simulink model "xieboduoji_13fangzhennow"  (R2023a)
settings: Solver=ode4  StartTime=0.0  StopTime=2.2  FixedStep=5e-7  RelTol=1e-3
undefined symbols (not defined in the file or in its folder): magnitude
libraries: simulink x417, spsRMSLib x70, spsCurrentMeasurementLib x32, spsVoltageMeasurementLib x31, powerlib_meascontrol x24, spsFourierLib x21, spsGroundLib x19, spsThreePhasePISectionLineLib x17, spsThreePhaseSeriesRLCBranchLib x14, spsdq0toAlphaBetaZeroLib x13, spsSeriesRLCBranchLib x11, spsUniversalBridgeLib x11
(part 2 of 12)

== system xieboduoji_13fangzhennow/node10/Subsystem2 ==
  u1 : Inport
  u3 : Inport  Port=2
  u4 : Inport  Port=3
  u5 : Inport  Port=4
  u6 : Inport  Port=5
  u2 : Inport  Port=6
  Pul : DiscretePulseGenerator  PulseType=Time based  Period=5e-5  PulseWidth=40
  RMS1 : Subsystem  TreatAsAtomicUnit=on
  k1 : Outport  VectorParamsAs1DForOutWhenUnconnected=off
  k2 : Outport  Port=2  VectorParamsAs1DForOutWhenUnconnected=off
  k3 : Outport  Port=3  VectorParamsAs1DForOutWhenUnconnected=off
  k4 : Outport  Port=4  VectorParamsAs1DForOutWhenUnconnected=off
  k5 : Outport  Port=5  VectorParamsAs1DForOutWhenUnconnected=off
  k6 : Outport  Port=6  VectorParamsAs1DForOutWhenUnconnected=off
  k7 : Outport  Port=7  VectorParamsAs1DForOutWhenUnconnected=off
  k8 : Outport  Port=8  VectorParamsAs1DForOutWhenUnconnected=off
  k9 : Outport  Port=9  VectorParamsAs1DForOutWhenUnconnected=off
  k10 : Outport  Port=10  VectorParamsAs1DForOutWhenUnconnected=off
  k11 : Outport  Port=11  VectorParamsAs1DForOutWhenUnconnected=off
  k12 : Outport  Port=12  VectorParamsAs1DForOutWhenUnconnected=off
  wires:
  Pul/1 -> RMS1/Trigger
  RMS1/1(k1) -> k1/1
  RMS1/2(k2) -> k2/1
  RMS1/3(k3) -> k3/1
  RMS1/4(k4) -> k4/1
  RMS1/5(k5) -> k5/1
  RMS1/6(k6) -> k6/1
  RMS1/7(k7) -> k7/1
  RMS1/8(k8) -> k8/1
  RMS1/9(k9) -> k9/1
  RMS1/10(k10) -> k10/1
  RMS1/11(k11) -> k11/1
  RMS1/12(k12) -> k12/1
  u1/1 -> RMS1/1(u1)
  u3/1 -> RMS1/2(u3)
  u4/1 -> RMS1/3(u4)
  u5/1 -> RMS1/4(u5)
  u6/1 -> RMS1/5(u6)
  u2/1 -> RMS1/6(u2)

== system xieboduoji_13fangzhennow/node10/谐波源 ==
  Current Measurement1 : spsCurrentMeasurementLib/Current Measurement  PhasorSimulation=off  OutputType=Complex  PSBequivalent=0
  Demux1 : Demux  Commented=on  Outputs=6
  Demux2 : Demux  Commented=on  Outputs=6
  Display{,1..23} (24 alike) : Display  Commented=on
  Scope : Scope  Commented=on
  Scope1 : Scope  Commented=on
  Series RLC Branch3 : spsSeriesRLCBranchLib/Series RLC Branch  LConnTagsString=__new0  RConnTagsString=__new0  BranchType=R  Resistance=33.94  Inductance=0.5e-3  SetiL0=off  InitialCurrent=0  Capacitance=1e-6  Setx0=off  InitialVoltage=0  Measurements=None
  Subsystem1 : Subsystem  Commented=on
  Subsystem2 : Subsystem  Commented=on
  Universal Bridge : spsUniversalBridgeLib/Universal Bridge  Arms=3  SnubberResistance=1e5  SnubberCapacitance=inf  Device=Diodes  Ron=1e-3  Lon=0  ForwardVoltages="[  0  0  ]"  ForwardVoltage=0  GTOparameters=[ 10e-6 , 20e-6 ]  IGBTparameters=[ 1e-6 , 2e-6 ]  Measurements=None  Measurements_2=None  converterType=Rectifier
  傅里叶分解 : spsFourierLib/Fourier  Commented=on  Freq=50  n=[5 7 11 13 17 19]  InInit=[0, 0]  Ts=0
  A : PMIOPort  Side=Left
  B : PMIOPort  Port=2  Side=Left
  C : PMIOPort  Port=3  Side=Left
  wires:
  傅里叶分解/1 -> Demux1/1, Scope/1
  傅里叶分解/2 -> Demux2/1, Scope1/1
  Current Measurement1/1 -> 傅里叶分解/1
  Subsystem2/5(k5) -> Display4/1
  Subsystem2/2(k2) -> Display1/1
  Subsystem2/12(k12) -> Display11/1
  Subsystem2/9(k9) -> Display8/1
  Subsystem2/8(k8) -> Display7/1
  Subsystem1/1(k1) -> Display12/1
  Subsystem1/7(k7) -> Display20/1
  Subsystem1/10(k10) -> Display23/1
  Subsystem1/3(k3) -> Display16/1
  Subsystem1/5(k5) -> Display18/1
  Subsystem2/11(k11) -> Display10/1
  Subsystem1/9(k9) -> Display22/1
  Subsystem1/11(k11) -> Display14/1
  Subsystem1/6(k6) -> Display19/1
  Subsystem1/2(k2) -> Display13/1
  Subsystem1/4(k4) -> Display17/1
  Subsystem1/12(k12) -> Display15/1
  Demux2/5 -> Subsystem1/5(u6)
  Demux2/4 -> Subsystem1/4(u5)
  Demux2/2 -> Subsystem1/2(u3)
  Demux2/6 -> Subsystem1/6(u2)
  Demux2/1 -> Subsystem1/1(u1)
  Subsystem2/6(k6) -> Display5/1
  Subsystem2/4(k4) -> Display3/1
  Subsystem2/7(k7) -> Display6/1
  Demux1/6 -> Subsystem2/6(u2)
  Demux1/5 -> Subsystem2/5(u6)
  Demux1/2 -> Subsystem2/2(u3)
  Demux1/4 -> Subsystem2/4(u5)
  Subsystem1/8(k8) -> Display21/1
  Subsystem2/10(k10) -> Display9/1
  Demux1/3 -> Subsystem2/3(u4)
  Subsystem2/3(k3) -> Display2/1
  Demux1/1 -> Subsystem2/1(u1)
  Demux2/3 -> Subsystem1/3(u4)
  Subsystem2/1(k1) -> Display/1
  connections:
  Universal Bridge/LConn3 -- C/RConn1
  Universal Bridge/RConn2 -- Series RLC Branch3/RConn1
  Universal Bridge/RConn1 -- Series RLC Branch3/LConn1
  Universal Bridge/LConn2 -- B/RConn1
  Current Measurement1/LConn1 -- Universal Bridge/LConn1
  A/RConn1 -- Current Measurement1/RConn1

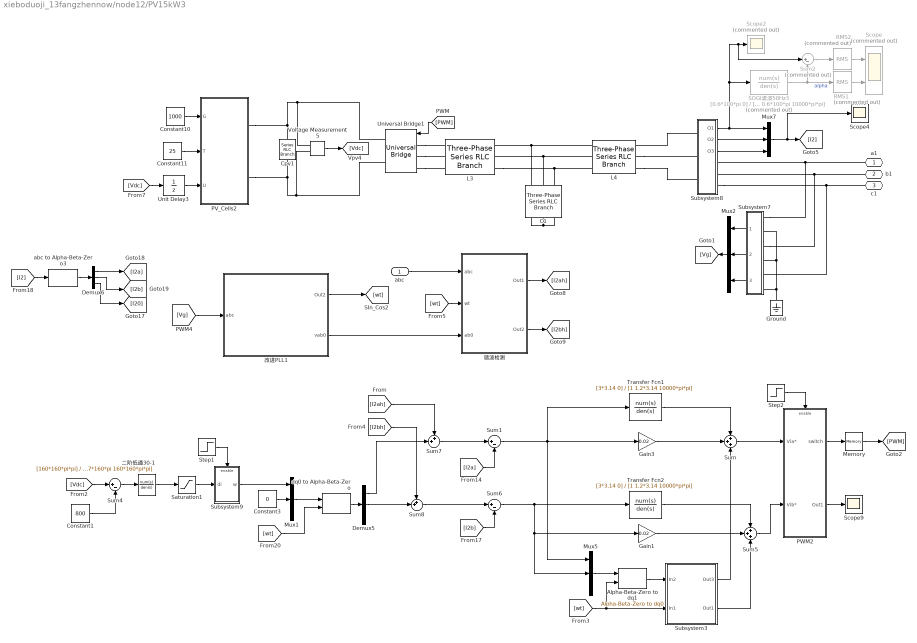
== system xieboduoji_13fangzhennow/node12/PV15kW3 ==
  abc : Inport
  " 二阶低通30-1" : TransferFcn  Numerator=[160*160*pi*pi]  Denominator=[1 2*0.707*160*pi 160*160*pi*pi]
  Alpha-Beta-Zero to dq1 : spsAlphaBetaZerotodq0Lib/Alpha-Beta-Zero to dq0  Alignment=90 degrees behind phase A axis
  C1 : spsThreePhaseSeriesRLCBranchLib/Three-Phase Series RLC Branch  LConnTagsString=A|B|C  RConnTagsString=A|B|C  BranchType=RC  Resistance=6  Inductance=1.5e-3  Capacitance=3e-6  Measurements=None
  Constant1 : Constant  Value=800
  Constant10 : Constant  Value=1000
  Constant11 : Constant  Value=25
  Constant3 : Constant  Value=0
  Cpv1 : spsSeriesRLCBranchLib/Series RLC Branch  LConnTagsString=__new0  RConnTagsString=__new0  BranchType=C  Resistance=0.2  Inductance=0.01e-3  SetiL0=off  InitialCurrent=0  Capacitance=2.5e-3  Setx0=on  InitialVoltage=800  Measurements=None
  Demux5 : Demux  Outputs=3
  Demux6 : Demux  Outputs=3
  Gain1 : Gain  Gain=0.02
  Gain3 : Gain  Gain=0.02
  Ground : spsGroundLib/Ground  LConnTagsString=a
  L3 : spsThreePhaseSeriesRLCBranchLib/Three-Phase Series RLC Branch  LConnTagsString=A|B|C  RConnTagsString=A|B|C  BranchType=L  Resistance=0.02  Inductance=2e-3  Capacitance=1e-6  Measurements=None
  L4 : spsThreePhaseSeriesRLCBranchLib/Three-Phase Series RLC Branch  LConnTagsString=A|B|C  RConnTagsString=A|B|C  BranchType=L  Resistance=0.02  Inductance=0.2e-3  Capacitance=1e-6  Measurements=None
  Memory : Memory
  Mux{1..2,5,7} (4 alike) : Mux  Inputs=3
  PV_Cells2 : Subsystem  mask{Parallel=1.6476, Series=30.3474}
  PWM2 : Subsystem
  RMS1 : spsRMSLib/RMS  Commented=on  TrueRMS=on  Freq=50  RMSInit=0  Ts=5e-5
  RMS2 : spsRMSLib/RMS  Commented=on  TrueRMS=on  Freq=50  RMSInit=0  Ts=5e-5
  SOGI滤波50Hz3 : TransferFcn  Commented=on  Numerator=[0.6*100*pi 0]  Denominator=[1 0.6*100*pi 10000*pi*pi]
  Saturation1 : Saturate  UpperLimit=15  LowerLimit=-15
  Scope : Scope  Commented=on  NumInputPorts=2
  Scope2 : Scope  Commented=on
  Scope4 : Scope
  Scope9 : Scope
  Step1 : Step  Time=0.4  SampleTime=0
  Step2 : Step  Time=0.4  SampleTime=0
  Subsystem3 : Subsystem
  Subsystem7 : Subsystem
  Subsystem8 : Subsystem
  Subsystem9 : Subsystem
  Sum : Sum  Inputs=+++
  Sum1 : Sum  Inputs=|+-
  Sum2 : Sum  Commented=on  Inputs=|+-
  Sum4 : Sum  Inputs=|+-
  Sum5 : Sum  Inputs=+++
  Sum6 : Sum  Inputs=|+-
  Sum7 : Sum  Inputs=++|
  Sum8 : Sum  Inputs=++|
  Transfer Fcn1 : TransferFcn  Numerator=[3*3.14 0]  Denominator=[1 1.2*3.14 10000*pi*pi]
  Transfer Fcn2 : TransferFcn  Numerator=[3*3.14 0]  Denominator=[1 1.2*3.14 10000*pi*pi]
  Unit Delay3 : UnitDelay  SampleTime=-1  HasFrameUpgradeWarning=on
  Universal Bridge1 : spsUniversalBridgeLib/Universal Bridge  Arms=3  SnubberResistance=1e5  SnubberCapacitance=inf  Device=IGBT / Diodes  Ron=0.002  Lon=0  ForwardVoltages="[  0  0  ]"  ForwardVoltage=0  GTOparameters=[ 10e-6 , 20e-6 ]  IGBTparameters=[ 1e-6 , 2e-6 ]  Measurements=None  Measurements_2=None  converterType=Rectifier
  Voltage Measurement5 : spsVoltageMeasurementLib/Voltage Measurement  PhasorSimulation=off  OutputType=Complex  PSBequivalent=0
  abc to Alpha-Beta-Zero3 : spsabctoAlphaBetaZeroLib/abc to Alpha-Beta-Zero
  dq0 to Alpha-Beta-Zero : spsdq0toAlphaBetaZeroLib/dq0 to Alpha-Beta-Zero  Alignment=Aligned with phase A axis
  改进PLL1 : Subsystem
  谐波检测 : Subsystem
  a1 : PMIOPort  Side=Right
  b1 : PMIOPort  Port=2  Side=Right
  c1 : PMIOPort  Port=3  Side=Right
  wires:
  Memory/1 -> [PWM]
  PWM2/2(Out1) -> Scope9/1
  Mux7/1 -> Scope4/1, [I2]
  [PWM] -> Universal Bridge1/1
  Subsystem8/3(O3) -> Mux7/3
  Subsystem8/2(O2) -> Mux7/2
  PWM2/1(switch) -> Memory/1
  Mux2/1 -> [Vg]
  Subsystem8/1(O1) -> Sum2/1, Scope2/1, SOGI滤波50Hz3/1, Mux7/1
  Subsystem7/1(O1) -> Mux2/1
  Subsystem7/2(O2) -> Mux2/2
  Subsystem7/3(O3) -> Mux2/3
  [I2b] -> Sum6/2
  Sum4/1 -> " 二阶低通30-1"/1
  Constant1/1 -> Sum4/2
  Mux1/1 -> dq0 to Alpha-Beta-Zero/1
  Sum1/1 -> Gain3/1, Transfer Fcn1/1, Mux5/1
  [wt] -> dq0 to Alpha-Beta-Zero/2
  dq0 to Alpha-Beta-Zero/1 -> Demux5/1
  Sum6/1 -> Gain1/1, Mux5/2, Transfer Fcn2/1
  [I2a] -> Sum1/2
  Sum7/1 -> Sum1/1
  Demux5/1 -> Sum7/2
  Demux5/2 -> Sum8/2
  Sum8/1 -> Sum6/1
  Subsystem9/1(w) -> Mux1/1
  Voltage Measurement5/1 -> [Vdc]
  Demux6/2 -> [I2b]
  Demux6/3 -> [I20]
  abc to Alpha-Beta-Zero3/1 -> Demux6/1
  Demux6/1 -> [I2a]
  [I2] -> abc to Alpha-Beta-Zero3/1
  Gain1/1 -> Sum5/2
  Gain3/1 -> Sum/2
  [Vdc] -> Sum4/1
  Alpha-Beta-Zero to dq1/1 -> Subsystem3/1(In2)
  [wt] -> Subsystem3/2(In1), Alpha-Beta-Zero to dq1/2
  Transfer Fcn1/1 -> Sum/1
  Transfer Fcn2/1 -> Sum5/1
  Mux5/1 -> Alpha-Beta-Zero to dq1/1
  Subsystem3/1(Out3) -> Sum/3
  Subsystem3/2(Out1) -> Sum5/3
  [Vg] -> 改进PLL1/1(abc)
  Constant3/1 -> Mux1/2
  [I2bh] -> Sum8/1
  [I2ah] -> Sum7/1
  Constant11/1 -> PV_Cells2/2(T)
  Constant10/1 -> PV_Cells2/1(G)
  Unit Delay3/1 -> PV_Cells2/3(U)
  [Vdc] -> Unit Delay3/1
  Step1/1 -> Subsystem9/Enable
  Saturation1/1 -> Subsystem9/1(di)
  " 二阶低通30-1"/1 -> Saturation1/1
  Step2/1 -> PWM2/Enable
  Sum/1 -> PWM2/1(Via*)
  Sum5/1 -> PWM2/2(Vib*)
  改进PLL1/1(Out2) -> [wt]
  谐波检测/2(Out2) -> [I2bh]
  [wt] -> 谐波检测/2(wt)
  abc/1 -> 谐波检测/1(abc)
  谐波检测/1(Out1) -> [I2ah]
  改进PLL1/2(vab0) -> 谐波检测/3(ab0)
  SOGI滤波50Hz3/1 -> RMS1/1, Sum2/2  "alpha"
  Sum2/1 -> RMS2/1
  RMS1/1 -> Scope/2
  RMS2/1 -> Scope/1
  connections:
  L4/RConn3 -- Subsystem8/LConn3
  C1/LConn1 -- L4/LConn1 -- L3/RConn1
  Subsystem8/LConn1 -- L4/RConn1
  Universal Bridge1/LConn1 -- L3/LConn1
  C1/LConn2 -- L4/LConn2 -- L3/RConn2
  Universal Bridge1/RConn1 -- Voltage Measurement5/LConn1 -- Cpv1/LConn1 -- PV_Cells2/RConn1
  Universal Bridge1/LConn2 -- L3/LConn2
  L4/RConn2 -- Subsystem8/LConn2
  Subsystem7/LConn3 -- b1/RConn1 -- Subsystem8/RConn2
  Universal Bridge1/LConn3 -- L3/LConn3
  L3/RConn3 -- C1/LConn3 -- L4/LConn3
  Subsystem7/LConn1 -- a1/RConn1 -- Subsystem8/RConn1
  Subsystem8/RConn3 -- c1/RConn1 -- Subsystem7/LConn5
  C1/RConn2 -- C1/RConn1 -- C1/RConn3
  Subsystem7/LConn2 -- Subsystem7/LConn4 -- Ground/LConn1 -- Subsystem7/LConn6
  Universal Bridge1/RConn2 -- Voltage Measurement5/LConn2 -- PV_Cells2/RConn2 -- Cpv1/RConn1

== system xieboduoji_13fangzhennow/node12/Subsystem1 ==
  u1 : Inport
  u3 : Inport  Port=2
  u4 : Inport  Port=3
  u5 : Inport  Port=4
  u6 : Inport  Port=5
  u2 : Inport  Port=6
  Pul : DiscretePulseGenerator  PulseType=Time based  Period=5e-5  PulseWidth=40
  RMS1 : Subsystem  TreatAsAtomicUnit=on
  k1 : Outport  VectorParamsAs1DForOutWhenUnconnected=off
  k2 : Outport  Port=2  VectorParamsAs1DForOutWhenUnconnected=off
  k3 : Outport  Port=3  VectorParamsAs1DForOutWhenUnconnected=off
  k4 : Outport  Port=4  VectorParamsAs1DForOutWhenUnconnected=off
  k5 : Outport  Port=5  VectorParamsAs1DForOutWhenUnconnected=off
  k6 : Outport  Port=6  VectorParamsAs1DForOutWhenUnconnected=off
  k7 : Outport  Port=7  VectorParamsAs1DForOutWhenUnconnected=off
  k8 : Outport  Port=8  VectorParamsAs1DForOutWhenUnconnected=off
  k9 : Outport  Port=9  VectorParamsAs1DForOutWhenUnconnected=off
  k10 : Outport  Port=10  VectorParamsAs1DForOutWhenUnconnected=off
  k11 : Outport  Port=11  VectorParamsAs1DForOutWhenUnconnected=off
  k12 : Outport  Port=12  VectorParamsAs1DForOutWhenUnconnected=off
  wires:
  u2/1 -> RMS1/6(u2)
  u6/1 -> RMS1/5(u6)
  u5/1 -> RMS1/4(u5)
  u4/1 -> RMS1/3(u4)
  u3/1 -> RMS1/2(u3)
  u1/1 -> RMS1/1(u1)
  RMS1/12(k12) -> k12/1
  RMS1/11(k11) -> k11/1
  RMS1/10(k10) -> k10/1
  RMS1/9(k9) -> k9/1
  RMS1/8(k8) -> k8/1
  RMS1/7(k7) -> k7/1
  RMS1/6(k6) -> k6/1
  RMS1/5(k5) -> k5/1
  RMS1/4(k4) -> k4/1
  RMS1/3(k3) -> k3/1
  RMS1/2(k2) -> k2/1
  RMS1/1(k1) -> k1/1
  Pul/1 -> RMS1/Trigger

== system xieboduoji_13fangzhennow/node12/Subsystem2 ==
  u1 : Inport
  u3 : Inport  Port=2
  u4 : Inport  Port=3
  u5 : Inport  Port=4
  u6 : Inport  Port=5
  u2 : Inport  Port=6
  Pul : DiscretePulseGenerator  PulseType=Time based  Period=5e-5  PulseWidth=40
  RMS1 : Subsystem  TreatAsAtomicUnit=on
  k1 : Outport  VectorParamsAs1DForOutWhenUnconnected=off
  k2 : Outport  Port=2  VectorParamsAs1DForOutWhenUnconnected=off
  k3 : Outport  Port=3  VectorParamsAs1DForOutWhenUnconnected=off
  k4 : Outport  Port=4  VectorParamsAs1DForOutWhenUnconnected=off
  k5 : Outport  Port=5  VectorParamsAs1DForOutWhenUnconnected=off
  k6 : Outport  Port=6  VectorParamsAs1DForOutWhenUnconnected=off
  k7 : Outport  Port=7  VectorParamsAs1DForOutWhenUnconnected=off
  k8 : Outport  Port=8  VectorParamsAs1DForOutWhenUnconnected=off
  k9 : Outport  Port=9  VectorParamsAs1DForOutWhenUnconnected=off
  k10 : Outport  Port=10  VectorParamsAs1DForOutWhenUnconnected=off
  k11 : Outport  Port=11  VectorParamsAs1DForOutWhenUnconnected=off
  k12 : Outport  Port=12  VectorParamsAs1DForOutWhenUnconnected=off
  wires:
  Pul/1 -> RMS1/Trigger
  RMS1/1(k1) -> k1/1
  RMS1/2(k2) -> k2/1
  RMS1/3(k3) -> k3/1
  RMS1/4(k4) -> k4/1
  RMS1/5(k5) -> k5/1
  RMS1/6(k6) -> k6/1
  RMS1/7(k7) -> k7/1
  RMS1/8(k8) -> k8/1
  RMS1/9(k9) -> k9/1
  RMS1/10(k10) -> k10/1
  RMS1/11(k11) -> k11/1
  RMS1/12(k12) -> k12/1
  u1/1 -> RMS1/1(u1)
  u3/1 -> RMS1/2(u3)
  u4/1 -> RMS1/3(u4)
  u5/1 -> RMS1/4(u5)
  u6/1 -> RMS1/5(u6)
  u2/1 -> RMS1/6(u2)

== system xieboduoji_13fangzhennow/node12/谐波源1 ==
  Current Measurement1 : spsCurrentMeasurementLib/Current Measurement  PhasorSimulation=off  OutputType=Complex  PSBequivalent=0
  Demux1 : Demux  Commented=on  Outputs=6
  Demux2 : Demux  Commented=on  Outputs=6
  Display{,1..23} (24 alike) : Display  Commented=on
  Scope : Scope  Commented=on
  Scope1 : Scope  Commented=on
  Series RLC Branch3 : spsSeriesRLCBranchLib/Series RLC Branch  LConnTagsString=__new0  RConnTagsString=__new0  BranchType=R  Resistance=24  Inductance=0.5e-3  SetiL0=off  InitialCurrent=0  Capacitance=1e-6  Setx0=off  InitialVoltage=0  Measurements=None
  Subsystem1 : Subsystem  Commented=on
  Subsystem2 : Subsystem  Commented=on
  Universal Bridge : spsUniversalBridgeLib/Universal Bridge  Arms=3  SnubberResistance=1e5  SnubberCapacitance=inf  Device=Diodes  Ron=1e-3  Lon=0  ForwardVoltages="[  0  0  ]"  ForwardVoltage=0  GTOparameters=[ 10e-6 , 20e-6 ]  IGBTparameters=[ 1e-6 , 2e-6 ]  Measurements=None  Measurements_2=None  converterType=Rectifier
  傅里叶分解 : spsFourierLib/Fourier  Commented=on  Freq=50  n=[5 7 11 13 17 19]  InInit=[0, 0]  Ts=0
  A : PMIOPort  Side=Left
  B : PMIOPort  Port=2  Side=Left
  C : PMIOPort  Port=3  Side=Left
  wires:
  傅里叶分解/1 -> Demux1/1, Scope/1
  傅里叶分解/2 -> Demux2/1, Scope1/1
  Current Measurement1/1 -> 傅里叶分解/1
  Subsystem2/5(k5) -> Display4/1
  Subsystem2/2(k2) -> Display1/1
  Subsystem2/12(k12) -> Display11/1
  Subsystem2/9(k9) -> Display8/1
  Subsystem2/8(k8) -> Display7/1
  Subsystem1/1(k1) -> Display12/1
  Subsystem1/7(k7) -> Display20/1
  Subsystem1/10(k10) -> Display23/1
  Subsystem1/3(k3) -> Display16/1
  Subsystem1/5(k5) -> Display18/1
  Subsystem2/11(k11) -> Display10/1
  Subsystem1/9(k9) -> Display22/1
  Subsystem1/11(k11) -> Display14/1
  Subsystem1/6(k6) -> Display19/1
  Subsystem1/2(k2) -> Display13/1
  Subsystem1/4(k4) -> Display17/1
  Subsystem1/12(k12) -> Display15/1
  Demux2/5 -> Subsystem1/5(u6)
  Demux2/4 -> Subsystem1/4(u5)
  Demux2/2 -> Subsystem1/2(u3)
  Demux2/6 -> Subsystem1/6(u2)
  Demux2/1 -> Subsystem1/1(u1)
  Subsystem2/6(k6) -> Display5/1
  Subsystem2/4(k4) -> Display3/1
  Subsystem2/7(k7) -> Display6/1
  Demux1/6 -> Subsystem2/6(u2)
  Demux1/5 -> Subsystem2/5(u6)
  Demux1/2 -> Subsystem2/2(u3)
  Demux1/4 -> Subsystem2/4(u5)
  Subsystem1/8(k8) -> Display21/1
  Subsystem2/10(k10) -> Display9/1
  Demux1/3 -> Subsystem2/3(u4)
  Subsystem2/3(k3) -> Display2/1
  Demux1/1 -> Subsystem2/1(u1)
  Demux2/3 -> Subsystem1/3(u4)
  Subsystem2/1(k1) -> Display/1
  connections:
  Universal Bridge/LConn3 -- C/RConn1
  Universal Bridge/RConn2 -- Series RLC Branch3/RConn1
  Universal Bridge/RConn1 -- Series RLC Branch3/LConn1
  Universal Bridge/LConn2 -- B/RConn1
  Current Measurement1/LConn1 -- Universal Bridge/LConn1
  A/RConn1 -- Current Measurement1/RConn1

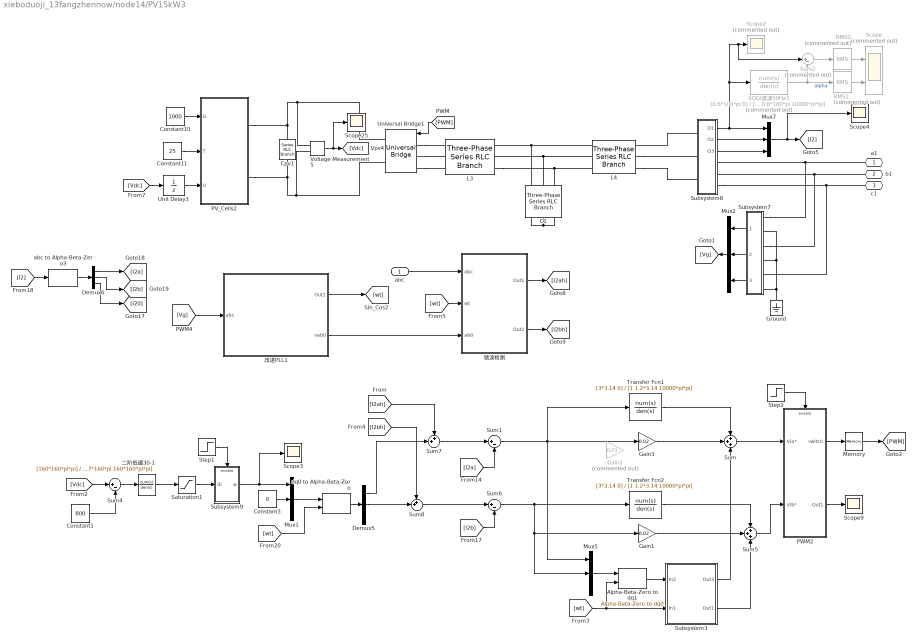
== system xieboduoji_13fangzhennow/node14/PV15kW3 ==
  abc : Inport
  " 二阶低通30-1" : TransferFcn  Numerator=[160*160*pi*pi]  Denominator=[1 2*0.707*160*pi 160*160*pi*pi]
  Alpha-Beta-Zero to dq1 : spsAlphaBetaZerotodq0Lib/Alpha-Beta-Zero to dq0  Alignment=90 degrees behind phase A axis
  C1 : spsThreePhaseSeriesRLCBranchLib/Three-Phase Series RLC Branch  LConnTagsString=A|B|C  RConnTagsString=A|B|C  BranchType=RC  Resistance=6  Inductance=1.5e-3  Capacitance=3e-6  Measurements=None
  Constant1 : Constant  Value=800
  Constant10 : Constant  Value=1000
  Constant11 : Constant  Value=25
  Constant3 : Constant  Value=0
  Cpv1 : spsSeriesRLCBranchLib/Series RLC Branch  LConnTagsString=__new0  RConnTagsString=__new0  BranchType=C  Resistance=0.2  Inductance=0.01e-3  SetiL0=off  InitialCurrent=0  Capacitance=2.5e-3  Setx0=on  InitialVoltage=800  Measurements=None
  Demux5 : Demux  Outputs=3
  Demux6 : Demux  Outputs=3
  Gain1 : Gain  Gain=0.02
  Gain2 : Gain  Commented=on  Gain=0.03
  Gain3 : Gain  Gain=0.02
  Ground : spsGroundLib/Ground  LConnTagsString=a
  L3 : spsThreePhaseSeriesRLCBranchLib/Three-Phase Series RLC Branch  LConnTagsString=A|B|C  RConnTagsString=A|B|C  BranchType=L  Resistance=0.02  Inductance=2e-3  Capacitance=1e-6  Measurements=None
  L4 : spsThreePhaseSeriesRLCBranchLib/Three-Phase Series RLC Branch  LConnTagsString=A|B|C  RConnTagsString=A|B|C  BranchType=L  Resistance=0.02  Inductance=0.2e-3  Capacitance=1e-6  Measurements=None
  Memory : Memory
  Mux{1..2,5,7} (4 alike) : Mux  Inputs=3
  PV_Cells2 : Subsystem  mask{Parallel=1.6476, Series=30.3474}
  PWM2 : Subsystem
  RMS1 : spsRMSLib/RMS  Commented=on  TrueRMS=on  Freq=50  RMSInit=0  Ts=5e-5
  RMS2 : spsRMSLib/RMS  Commented=on  TrueRMS=on  Freq=50  RMSInit=0  Ts=5e-5
  SOGI滤波50Hz3 : TransferFcn  Commented=on  Numerator=[0.6*100*pi 0]  Denominator=[1 0.6*100*pi 10000*pi*pi]
  Saturation1 : Saturate  UpperLimit=15  LowerLimit=-15
  Scope : Scope  Commented=on  NumInputPorts=2
  Scope2 : Scope  Commented=on
  Scope{3..4,9,25} (4 alike) : Scope
  Step1 : Step  Time=0.4  SampleTime=0
  Step2 : Step  Time=0.4  SampleTime=0
  Subsystem3 : Subsystem
  Subsystem7 : Subsystem
  Subsystem8 : Subsystem
  Subsystem9 : Subsystem
  Sum : Sum  Inputs=+++
  Sum1 : Sum  Inputs=|+-
  Sum2 : Sum  Commented=on  Inputs=|+-
  Sum4 : Sum  Inputs=|+-
  Sum5 : Sum  Inputs=+++
  Sum6 : Sum  Inputs=|+-
  Sum7 : Sum  Inputs=++|
  Sum8 : Sum  Inputs=++|
  Transfer Fcn1 : TransferFcn  Numerator=[3*3.14 0]  Denominator=[1 1.2*3.14 10000*pi*pi]
  Transfer Fcn2 : TransferFcn  Numerator=[3*3.14 0]  Denominator=[1 1.2*3.14 10000*pi*pi]
  Unit Delay3 : UnitDelay  SampleTime=-1  HasFrameUpgradeWarning=on
  Universal Bridge1 : spsUniversalBridgeLib/Universal Bridge  Arms=3  SnubberResistance=1e5  SnubberCapacitance=inf  Device=IGBT / Diodes  Ron=0.002  Lon=0  ForwardVoltages="[  0  0  ]"  ForwardVoltage=0  GTOparameters=[ 10e-6 , 20e-6 ]  IGBTparameters=[ 1e-6 , 2e-6 ]  Measurements=None  Measurements_2=None  converterType=Rectifier
  Voltage Measurement5 : spsVoltageMeasurementLib/Voltage Measurement  PhasorSimulation=off  OutputType=Complex  PSBequivalent=0
  abc to Alpha-Beta-Zero3 : spsabctoAlphaBetaZeroLib/abc to Alpha-Beta-Zero
  dq0 to Alpha-Beta-Zero : spsdq0toAlphaBetaZeroLib/dq0 to Alpha-Beta-Zero  Alignment=Aligned with phase A axis
  改进PLL1 : Subsystem
  谐波检测 : Subsystem
  a1 : PMIOPort  Side=Right
  b1 : PMIOPort  Port=2  Side=Right
  c1 : PMIOPort  Port=3  Side=Right
  wires:
  Memory/1 -> [PWM]
  PWM2/2(Out1) -> Scope9/1
  Mux7/1 -> Scope4/1, [I2]
  [PWM] -> Universal Bridge1/1
  Subsystem8/3(O3) -> Mux7/3
  Subsystem8/2(O2) -> Mux7/2
  PWM2/1(switch) -> Memory/1
  Mux2/1 -> [Vg]
  Subsystem8/1(O1) -> Sum2/1, Scope2/1, SOGI滤波50Hz3/1, Mux7/1
  Subsystem7/1(O1) -> Mux2/1
  Subsystem7/2(O2) -> Mux2/2
  Subsystem7/3(O3) -> Mux2/3
  [I2b] -> Sum6/2
  Sum4/1 -> " 二阶低通30-1"/1
  Constant1/1 -> Sum4/2
  Mux1/1 -> dq0 to Alpha-Beta-Zero/1
  Sum1/1 -> Gain3/1, Transfer Fcn1/1, Mux5/1
  [wt] -> dq0 to Alpha-Beta-Zero/2
  dq0 to Alpha-Beta-Zero/1 -> Demux5/1
  Sum6/1 -> Gain1/1, Mux5/2, Transfer Fcn2/1
  [I2a] -> Sum1/2
  Sum7/1 -> Sum1/1
  Demux5/1 -> Sum7/2
  Demux5/2 -> Sum8/2
  Sum8/1 -> Sum6/1
  Subsystem9/1(w) -> Mux1/1, Scope3/1
  Voltage Measurement5/1 -> Scope25/1, [Vdc]
  Demux6/2 -> [I2b]
  Demux6/3 -> [I20]
  abc to Alpha-Beta-Zero3/1 -> Demux6/1
  Demux6/1 -> [I2a]
  [I2] -> abc to Alpha-Beta-Zero3/1
  Gain1/1 -> Sum5/2
  Gain3/1 -> Sum/2
  [Vdc] -> Sum4/1
  Alpha-Beta-Zero to dq1/1 -> Subsystem3/1(In2)
  [wt] -> Subsystem3/2(In1), Alpha-Beta-Zero to dq1/2
  Transfer Fcn1/1 -> Sum/1
  Transfer Fcn2/1 -> Sum5/1
  Mux5/1 -> Alpha-Beta-Zero to dq1/1
  Subsystem3/1(Out3) -> Sum/3
  Subsystem3/2(Out1) -> Sum5/3
  [Vg] -> 改进PLL1/1(abc)
  Constant3/1 -> Mux1/2
  [I2bh] -> Sum8/1
  [I2ah] -> Sum7/1
  Constant11/1 -> PV_Cells2/2(T)
  Constant10/1 -> PV_Cells2/1(G)
  Unit Delay3/1 -> PV_Cells2/3(U)
  [Vdc] -> Unit Delay3/1
  Step1/1 -> Subsystem9/Enable
  Saturation1/1 -> Subsystem9/1(di)
  " 二阶低通30-1"/1 -> Saturation1/1
  Step2/1 -> PWM2/Enable
  Sum/1 -> PWM2/1(Via*)
  Sum5/1 -> PWM2/2(Vib*)
  改进PLL1/1(Out2) -> [wt]
  谐波检测/2(Out2) -> [I2bh]
  [wt] -> 谐波检测/2(wt)
  abc/1 -> 谐波检测/1(abc)
  谐波检测/1(Out1) -> [I2ah]
  改进PLL1/2(vab0) -> 谐波检测/3(ab0)
  SOGI滤波50Hz3/1 -> RMS1/1, Sum2/2  "alpha"
  Sum2/1 -> RMS2/1
  RMS1/1 -> Scope/2
  RMS2/1 -> Scope/1
  connections:
  L4/RConn3 -- Subsystem8/LConn3
  C1/LConn1 -- L4/LConn1 -- L3/RConn1
  Subsystem8/LConn1 -- L4/RConn1
  Universal Bridge1/LConn1 -- L3/LConn1
  C1/LConn2 -- L4/LConn2 -- L3/RConn2
  Universal Bridge1/RConn1 -- Voltage Measurement5/LConn1 -- Cpv1/LConn1 -- PV_Cells2/RConn1
  Universal Bridge1/LConn2 -- L3/LConn2
  L4/RConn2 -- Subsystem8/LConn2
  Subsystem7/LConn3 -- b1/RConn1 -- Subsystem8/RConn2
  Universal Bridge1/LConn3 -- L3/LConn3
  L3/RConn3 -- C1/LConn3 -- L4/LConn3
  Subsystem7/LConn1 -- a1/RConn1 -- Subsystem8/RConn1
  Subsystem8/RConn3 -- c1/RConn1 -- Subsystem7/LConn5
  C1/RConn2 -- C1/RConn1 -- C1/RConn3
  Subsystem7/LConn2 -- Subsystem7/LConn4 -- Ground/LConn1 -- Subsystem7/LConn6
  Universal Bridge1/RConn2 -- Voltage Measurement5/LConn2 -- PV_Cells2/RConn2 -- Cpv1/RConn1

== system xieboduoji_13fangzhennow/node14/Subsystem1 ==
  u1 : Inport
  u3 : Inport  Port=2
  u4 : Inport  Port=3
  u5 : Inport  Port=4
  u6 : Inport  Port=5
  u2 : Inport  Port=6
  Pul : DiscretePulseGenerator  PulseType=Time based  Period=5e-5  PulseWidth=40
  RMS1 : Subsystem  TreatAsAtomicUnit=on
  k1 : Outport  VectorParamsAs1DForOutWhenUnconnected=off
  k2 : Outport  Port=2  VectorParamsAs1DForOutWhenUnconnected=off
  k3 : Outport  Port=3  VectorParamsAs1DForOutWhenUnconnected=off
  k4 : Outport  Port=4  VectorParamsAs1DForOutWhenUnconnected=off
  k5 : Outport  Port=5  VectorParamsAs1DForOutWhenUnconnected=off
  k6 : Outport  Port=6  VectorParamsAs1DForOutWhenUnconnected=off
  k7 : Outport  Port=7  VectorParamsAs1DForOutWhenUnconnected=off
  k8 : Outport  Port=8  VectorParamsAs1DForOutWhenUnconnected=off
  k9 : Outport  Port=9  VectorParamsAs1DForOutWhenUnconnected=off
  k10 : Outport  Port=10  VectorParamsAs1DForOutWhenUnconnected=off
  k11 : Outport  Port=11  VectorParamsAs1DForOutWhenUnconnected=off
  k12 : Outport  Port=12  VectorParamsAs1DForOutWhenUnconnected=off
  wires:
  u2/1 -> RMS1/6(u2)
  u6/1 -> RMS1/5(u6)
  u5/1 -> RMS1/4(u5)
  u4/1 -> RMS1/3(u4)
  u3/1 -> RMS1/2(u3)
  u1/1 -> RMS1/1(u1)
  RMS1/12(k12) -> k12/1
  RMS1/11(k11) -> k11/1
  RMS1/10(k10) -> k10/1
  RMS1/9(k9) -> k9/1
  RMS1/8(k8) -> k8/1
  RMS1/7(k7) -> k7/1
  RMS1/6(k6) -> k6/1
  RMS1/5(k5) -> k5/1
  RMS1/4(k4) -> k4/1
  RMS1/3(k3) -> k3/1
  RMS1/2(k2) -> k2/1
  RMS1/1(k1) -> k1/1
  Pul/1 -> RMS1/Trigger

== system xieboduoji_13fangzhennow/node14/Subsystem2 ==
  u1 : Inport
  u3 : Inport  Port=2
  u4 : Inport  Port=3
  u5 : Inport  Port=4
  u6 : Inport  Port=5
  u2 : Inport  Port=6
  Pul : DiscretePulseGenerator  PulseType=Time based  Period=5e-5  PulseWidth=40
  RMS1 : Subsystem  TreatAsAtomicUnit=on
  k1 : Outport  VectorParamsAs1DForOutWhenUnconnected=off
  k2 : Outport  Port=2  VectorParamsAs1DForOutWhenUnconnected=off
  k3 : Outport  Port=3  VectorParamsAs1DForOutWhenUnconnected=off
  k4 : Outport  Port=4  VectorParamsAs1DForOutWhenUnconnected=off
  k5 : Outport  Port=5  VectorParamsAs1DForOutWhenUnconnected=off
  k6 : Outport  Port=6  VectorParamsAs1DForOutWhenUnconnected=off
  k7 : Outport  Port=7  VectorParamsAs1DForOutWhenUnconnected=off
  k8 : Outport  Port=8  VectorParamsAs1DForOutWhenUnconnected=off
  k9 : Outport  Port=9  VectorParamsAs1DForOutWhenUnconnected=off
  k10 : Outport  Port=10  VectorParamsAs1DForOutWhenUnconnected=off
  k11 : Outport  Port=11  VectorParamsAs1DForOutWhenUnconnected=off
  k12 : Outport  Port=12  VectorParamsAs1DForOutWhenUnconnected=off
  wires:
  Pul/1 -> RMS1/Trigger
  RMS1/1(k1) -> k1/1
  RMS1/2(k2) -> k2/1
  RMS1/3(k3) -> k3/1
  RMS1/4(k4) -> k4/1
  RMS1/5(k5) -> k5/1
  RMS1/6(k6) -> k6/1
  RMS1/7(k7) -> k7/1
  RMS1/8(k8) -> k8/1
  RMS1/9(k9) -> k9/1
  RMS1/10(k10) -> k10/1
  RMS1/11(k11) -> k11/1
  RMS1/12(k12) -> k12/1
  u1/1 -> RMS1/1(u1)
  u3/1 -> RMS1/2(u3)
  u4/1 -> RMS1/3(u4)
  u5/1 -> RMS1/4(u5)
  u6/1 -> RMS1/5(u6)
  u2/1 -> RMS1/6(u2)

== system xieboduoji_13fangzhennow/node14/谐波源 ==
  Current Measurement1 : spsCurrentMeasurementLib/Current Measurement  PhasorSimulation=off  OutputType=Complex  PSBequivalent=0
  Demux1 : Demux  Commented=on  Outputs=6
  Demux2 : Demux  Commented=on  Outputs=6
  Display{,1..23} (24 alike) : Display  Commented=on
  Scope : Scope  Commented=on
  Scope1 : Scope  Commented=on
  Series RLC Branch3 : spsSeriesRLCBranchLib/Series RLC Branch  LConnTagsString=__new0  RConnTagsString=__new0  BranchType=R  Resistance=33.94  Inductance=0.5e-3  SetiL0=off  InitialCurrent=0  Capacitance=1e-6  Setx0=off  InitialVoltage=0  Measurements=None
  Subsystem1 : Subsystem  Commented=on
  Subsystem2 : Subsystem  Commented=on
  Universal Bridge : spsUniversalBridgeLib/Universal Bridge  Arms=3  SnubberResistance=1e5  SnubberCapacitance=inf  Device=Diodes  Ron=1e-3  Lon=0  ForwardVoltages="[  0  0  ]"  ForwardVoltage=0  GTOparameters=[ 10e-6 , 20e-6 ]  IGBTparameters=[ 1e-6 , 2e-6 ]  Measurements=None  Measurements_2=None  converterType=Rectifier
  傅里叶分解 : spsFourierLib/Fourier  Commented=on  Freq=50  n=[5 7 11 13 17 19]  InInit=[0, 0]  Ts=0
  A : PMIOPort  Side=Left
  B : PMIOPort  Port=2  Side=Left
  C : PMIOPort  Port=3  Side=Left
  wires:
  傅里叶分解/1 -> Demux1/1, Scope/1
  傅里叶分解/2 -> Demux2/1, Scope1/1
  Current Measurement1/1 -> 傅里叶分解/1
  Subsystem2/5(k5) -> Display4/1
  Subsystem2/2(k2) -> Display1/1
  Subsystem2/12(k12) -> Display11/1
  Subsystem2/9(k9) -> Display8/1
  Subsystem2/8(k8) -> Display7/1
  Subsystem1/1(k1) -> Display12/1
  Subsystem1/7(k7) -> Display20/1
  Subsystem1/10(k10) -> Display23/1
  Subsystem1/3(k3) -> Display16/1
  Subsystem1/5(k5) -> Display18/1
  Subsystem2/11(k11) -> Display10/1
  Subsystem1/9(k9) -> Display22/1
  Subsystem1/11(k11) -> Display14/1
  Subsystem1/6(k6) -> Display19/1
  Subsystem1/2(k2) -> Display13/1
  Subsystem1/4(k4) -> Display17/1
  Subsystem1/12(k12) -> Display15/1
  Demux2/5 -> Subsystem1/5(u6)
  Demux2/4 -> Subsystem1/4(u5)
  Demux2/2 -> Subsystem1/2(u3)
  Demux2/6 -> Subsystem1/6(u2)
  Demux2/1 -> Subsystem1/1(u1)
  Subsystem2/6(k6) -> Display5/1
  Subsystem2/4(k4) -> Display3/1
  Subsystem2/7(k7) -> Display6/1
  Demux1/6 -> Subsystem2/6(u2)
  Demux1/5 -> Subsystem2/5(u6)
  Demux1/2 -> Subsystem2/2(u3)
  Demux1/4 -> Subsystem2/4(u5)
  Subsystem1/8(k8) -> Display21/1
  Subsystem2/10(k10) -> Display9/1
  Demux1/3 -> Subsystem2/3(u4)
  Subsystem2/3(k3) -> Display2/1
  Demux1/1 -> Subsystem2/1(u1)
  Demux2/3 -> Subsystem1/3(u4)
  Subsystem2/1(k1) -> Display/1
  connections:
  Universal Bridge/LConn3 -- C/RConn1
  Universal Bridge/RConn2 -- Series RLC Branch3/RConn1
  Universal Bridge/RConn1 -- Series RLC Branch3/LConn1
  Universal Bridge/LConn2 -- B/RConn1
  Current Measurement1/LConn1 -- Universal Bridge/LConn1
  A/RConn1 -- Current Measurement1/RConn1

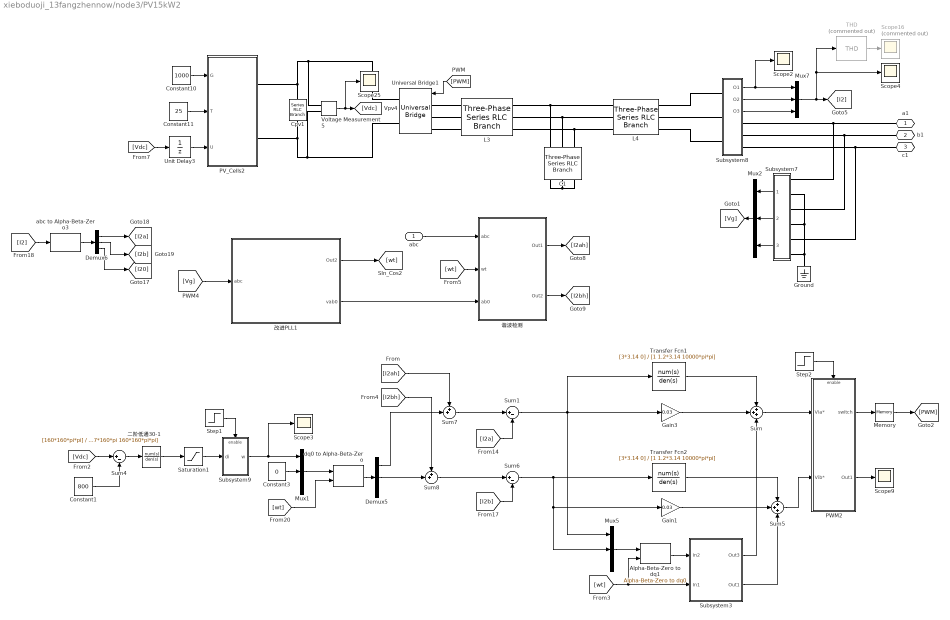
== system xieboduoji_13fangzhennow/node3/PV15kW2 ==
  abc : Inport
  " 二阶低通30-1" : TransferFcn  Numerator=[160*160*pi*pi]  Denominator=[1 2*0.707*160*pi 160*160*pi*pi]
  Alpha-Beta-Zero to dq1 : powerlib_meascontrol/Transformations/Alpha-Beta-Zero to dq0  Alignment=90 degrees behind phase A axis
  C1 : spsThreePhaseSeriesRLCBranchLib/Three-Phase Series RLC Branch  LConnTagsString=A|B|C  RConnTagsString=A|B|C  BranchType=RC  Resistance=6  Inductance=1.5e-3  Capacitance=3e-6  Measurements=None
  Constant1 : Constant  Value=800
  Constant10 : Constant  Value=1000
  Constant11 : Constant  Value=25
  Constant3 : Constant  Value=0
  Cpv1 : spsSeriesRLCBranchLib/Series RLC Branch  LConnTagsString=__new0  RConnTagsString=__new0  BranchType=C  Resistance=0.2  Inductance=0.01e-3  SetiL0=off  InitialCurrent=0  Capacitance=2.5e-3  Setx0=on  InitialVoltage=800  Measurements=None
  Demux5 : Demux  Outputs=3
  Demux6 : Demux  Outputs=3
  Gain1 : Gain  Gain=0.03
  Gain3 : Gain  Gain=0.03
  Ground : spsGroundLib/Ground  LConnTagsString=a
  L3 : spsThreePhaseSeriesRLCBranchLib/Three-Phase Series RLC Branch  LConnTagsString=A|B|C  RConnTagsString=A|B|C  BranchType=L  Resistance=0.02  Inductance=2e-3  Capacitance=1e-6  Measurements=None
  L4 : spsThreePhaseSeriesRLCBranchLib/Three-Phase Series RLC Branch  LConnTagsString=A|B|C  RConnTagsString=A|B|C  BranchType=L  Resistance=0.02  Inductance=0.2e-3  Capacitance=1e-6  Measurements=None
  Memory : Memory
  Mux{1..2,5,7} (4 alike) : Mux  Inputs=3
  PV_Cells2 : Subsystem  mask{Parallel=1.6476, Series=30.3474}
  PWM2 : Subsystem
  Saturation1 : Saturate  UpperLimit=15  LowerLimit=-15
  Scope16 : Scope  Commented=on
  Scope{2..4,9,25} (5 alike) : Scope
  Step1 : Step  Time=0.4  SampleTime=0
  Step2 : Step  Time=0.4  SampleTime=0
  Subsystem3 : Subsystem
  Subsystem7 : Subsystem
  Subsystem8 : Subsystem
  Subsystem9 : Subsystem
  Sum : Sum  Inputs=+++
  Sum1 : Sum  Inputs=|+-
  Sum4 : Sum  Inputs=|+-
  Sum5 : Sum  Inputs=+++
  Sum6 : Sum  Inputs=|+-
  Sum7 : Sum  Inputs=++|
  Sum8 : Sum  Inputs=++|
  THD : powerlib_meascontrol/Measurements/THD  Commented=on  Freq=50  Ts=0
  Transfer Fcn1 : TransferFcn  Numerator=[3*3.14 0]  Denominator=[1 1.2*3.14 10000*pi*pi]
  Transfer Fcn2 : TransferFcn  Numerator=[3*3.14 0]  Denominator=[1 1.2*3.14 10000*pi*pi]
  Unit Delay3 : UnitDelay  SampleTime=-1  HasFrameUpgradeWarning=on
  Universal Bridge1 : spsUniversalBridgeLib/Universal Bridge  Arms=3  SnubberResistance=1e5  SnubberCapacitance=inf  Device=IGBT / Diodes  Ron=0.002  Lon=0  ForwardVoltages="[  0  0  ]"  ForwardVoltage=0  GTOparameters=[ 10e-6 , 20e-6 ]  IGBTparameters=[ 1e-6 , 2e-6 ]  Measurements=None  Measurements_2=None  converterType=Rectifier
  Voltage Measurement5 : spsVoltageMeasurementLib/Voltage Measurement  PhasorSimulation=off  OutputType=Complex  PSBequivalent=0
  abc to Alpha-Beta-Zero3 : powerlib_meascontrol/Transformations/abc to Alpha-Beta-Zero
  dq0 to Alpha-Beta-Zero : powerlib_meascontrol/Transformations/dq0 to Alpha-Beta-Zero  Alignment=Aligned with phase A axis
  改进PLL1 : Subsystem
  谐波检测 : Subsystem
  a1 : PMIOPort  Side=Right
  b1 : PMIOPort  Port=2  Side=Right
  c1 : PMIOPort  Port=3  Side=Right
  wires:
  Memory/1 -> [PWM]
  PWM2/2(Out1) -> Scope9/1
  Mux7/1 -> THD/1, Scope4/1, [I2]
  [PWM] -> Universal Bridge1/1
  Subsystem8/3(O3) -> Mux7/3
  Subsystem8/2(O2) -> Mux7/2
  PWM2/1(switch) -> Memory/1
  Mux2/1 -> [Vg]
  Subsystem8/1(O1) -> Scope2/1, Mux7/1
  Subsystem7/1(O1) -> Mux2/1
  Subsystem7/2(O2) -> Mux2/2
  Subsystem7/3(O3) -> Mux2/3
  [I2b] -> Sum6/2
  Sum4/1 -> " 二阶低通30-1"/1
  Constant1/1 -> Sum4/2
  Mux1/1 -> dq0 to Alpha-Beta-Zero/1
  Sum1/1 -> Gain3/1, Transfer Fcn1/1, Mux5/1
  [wt] -> dq0 to Alpha-Beta-Zero/2
  dq0 to Alpha-Beta-Zero/1 -> Demux5/1
  Sum6/1 -> Gain1/1, Mux5/2, Transfer Fcn2/1
  [I2a] -> Sum1/2
  Sum7/1 -> Sum1/1
  Demux5/1 -> Sum7/2
  Demux5/2 -> Sum8/2
  Sum8/1 -> Sum6/1
  Subsystem9/1(w) -> Mux1/1, Scope3/1
  THD/1 -> Scope16/1
  Voltage Measurement5/1 -> Scope25/1, [Vdc]
  Demux6/2 -> [I2b]
  Demux6/3 -> [I20]
  abc to Alpha-Beta-Zero3/1 -> Demux6/1
  Demux6/1 -> [I2a]
  [I2] -> abc to Alpha-Beta-Zero3/1
  Gain1/1 -> Sum5/2
  Gain3/1 -> Sum/2
  [Vdc] -> Sum4/1
  Alpha-Beta-Zero to dq1/1 -> Subsystem3/1(In2)
  [wt] -> Subsystem3/2(In1), Alpha-Beta-Zero to dq1/2
  Transfer Fcn1/1 -> Sum/1
  Transfer Fcn2/1 -> Sum5/1
  Mux5/1 -> Alpha-Beta-Zero to dq1/1
  Subsystem3/1(Out3) -> Sum/3
  Subsystem3/2(Out1) -> Sum5/3
  [Vg] -> 改进PLL1/1(abc)
  Constant3/1 -> Mux1/2
  [I2bh] -> Sum8/1
  [I2ah] -> Sum7/1
  Constant11/1 -> PV_Cells2/2(T)
  Constant10/1 -> PV_Cells2/1(G)
  Unit Delay3/1 -> PV_Cells2/3(U)
  [Vdc] -> Unit Delay3/1
  Step1/1 -> Subsystem9/Enable
  Saturation1/1 -> Subsystem9/1(di)
  " 二阶低通30-1"/1 -> Saturation1/1
  Step2/1 -> PWM2/Enable
  Sum/1 -> PWM2/1(Via*)
  Sum5/1 -> PWM2/2(Vib*)
  改进PLL1/1(Out2) -> [wt]
  谐波检测/2(Out2) -> [I2bh]
  [wt] -> 谐波检测/2(wt)
  abc/1 -> 谐波检测/1(abc)
  谐波检测/1(Out1) -> [I2ah]
  改进PLL1/2(vab0) -> 谐波检测/3(ab0)
  connections:
  L4/RConn3 -- Subsystem8/LConn3
  C1/LConn1 -- L4/LConn1 -- L3/RConn1
  Subsystem8/LConn1 -- L4/RConn1
  Universal Bridge1/LConn1 -- L3/LConn1
  C1/LConn2 -- L4/LConn2 -- L3/RConn2
  Universal Bridge1/RConn1 -- Voltage Measurement5/LConn1 -- Cpv1/LConn1 -- PV_Cells2/RConn1
  Universal Bridge1/LConn2 -- L3/LConn2
  L4/RConn2 -- Subsystem8/LConn2
  Subsystem7/LConn3 -- b1/RConn1 -- Subsystem8/RConn2
  Universal Bridge1/LConn3 -- L3/LConn3
  L3/RConn3 -- C1/LConn3 -- L4/LConn3
  Subsystem7/LConn1 -- a1/RConn1 -- Subsystem8/RConn1
  Subsystem8/RConn3 -- c1/RConn1 -- Subsystem7/LConn5
  C1/RConn2 -- C1/RConn1 -- C1/RConn3
  Subsystem7/LConn2 -- Subsystem7/LConn4 -- Ground/LConn1 -- Subsystem7/LConn6
  Universal Bridge1/RConn2 -- Voltage Measurement5/LConn2 -- PV_Cells2/RConn2 -- Cpv1/RConn1

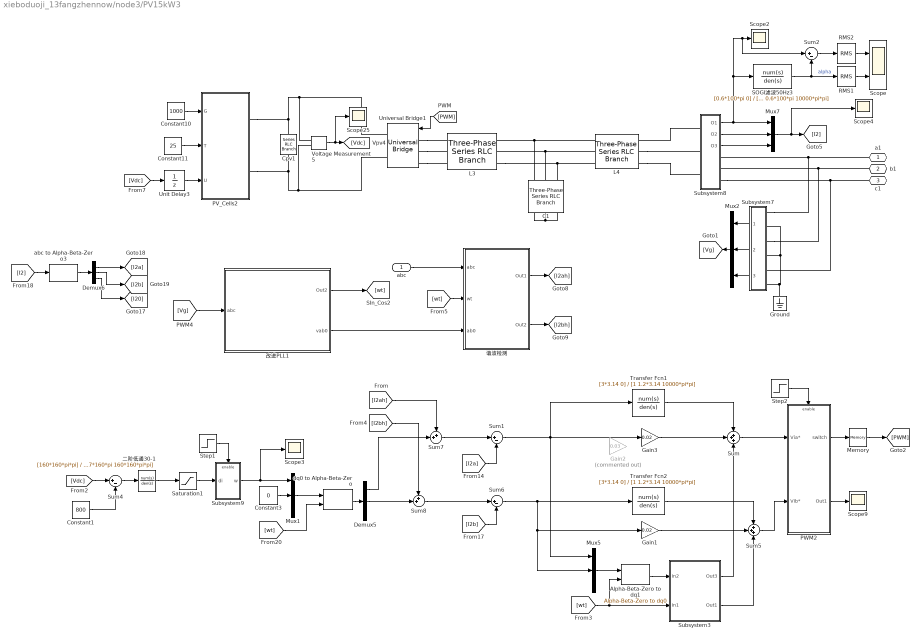
== system xieboduoji_13fangzhennow/node3/PV15kW3 ==
  abc : Inport
  " 二阶低通30-1" : TransferFcn  Numerator=[160*160*pi*pi]  Denominator=[1 2*0.707*160*pi 160*160*pi*pi]
  Alpha-Beta-Zero to dq1 : spsAlphaBetaZerotodq0Lib/Alpha-Beta-Zero to dq0  Alignment=90 degrees behind phase A axis
  C1 : spsThreePhaseSeriesRLCBranchLib/Three-Phase Series RLC Branch  LConnTagsString=A|B|C  RConnTagsString=A|B|C  BranchType=RC  Resistance=6  Inductance=1.5e-3  Capacitance=3e-6  Measurements=None
  Constant1 : Constant  Value=800
  Constant10 : Constant  Value=1000
  Constant11 : Constant  Value=25
  Constant3 : Constant  Value=0
  Cpv1 : spsSeriesRLCBranchLib/Series RLC Branch  LConnTagsString=__new0  RConnTagsString=__new0  BranchType=C  Resistance=0.2  Inductance=0.01e-3  SetiL0=off  InitialCurrent=0  Capacitance=2.5e-3  Setx0=on  InitialVoltage=800  Measurements=None
  Demux5 : Demux  Outputs=3
  Demux6 : Demux  Outputs=3
  Gain1 : Gain  Gain=0.02
  Gain2 : Gain  Commented=on  Gain=0.03
  Gain3 : Gain  Gain=0.02
  Ground : spsGroundLib/Ground  LConnTagsString=a
  L3 : spsThreePhaseSeriesRLCBranchLib/Three-Phase Series RLC Branch  LConnTagsString=A|B|C  RConnTagsString=A|B|C  BranchType=L  Resistance=0.02  Inductance=2e-3  Capacitance=1e-6  Measurements=None
  L4 : spsThreePhaseSeriesRLCBranchLib/Three-Phase Series RLC Branch  LConnTagsString=A|B|C  RConnTagsString=A|B|C  BranchType=L  Resistance=0.02  Inductance=0.2e-3  Capacitance=1e-6  Measurements=None
  Memory : Memory
  Mux{1..2,5,7} (4 alike) : Mux  Inputs=3
  PV_Cells2 : Subsystem  mask{Parallel=1.6476, Series=30.3474}
  PWM2 : Subsystem
  RMS1 : spsRMSLib/RMS  TrueRMS=on  Freq=50  RMSInit=0  Ts=5e-5
  RMS2 : spsRMSLib/RMS  TrueRMS=on  Freq=50  RMSInit=0  Ts=5e-5
  SOGI滤波50Hz3 : TransferFcn  Numerator=[0.6*100*pi 0]  Denominator=[1 0.6*100*pi 10000*pi*pi]
  Saturation1 : Saturate  UpperLimit=15  LowerLimit=-15
  Scope : Scope  NumInputPorts=2
  Scope{2..4,9,25} (5 alike) : Scope
  Step1 : Step  Time=0.4  SampleTime=0
  Step2 : Step  Time=0.4  SampleTime=0
  Subsystem3 : Subsystem
  Subsystem7 : Subsystem
  Subsystem8 : Subsystem
  Subsystem9 : Subsystem
  Sum : Sum  Inputs=+++
  Sum{1..2,4,6} (4 alike) : Sum  Inputs=|+-
  Sum5 : Sum  Inputs=+++
  Sum7 : Sum  Inputs=++|
  Sum8 : Sum  Inputs=++|
  Transfer Fcn1 : TransferFcn  Numerator=[3*3.14 0]  Denominator=[1 1.2*3.14 10000*pi*pi]
  Transfer Fcn2 : TransferFcn  Numerator=[3*3.14 0]  Denominator=[1 1.2*3.14 10000*pi*pi]
  Unit Delay3 : UnitDelay  SampleTime=-1  HasFrameUpgradeWarning=on
  Universal Bridge1 : spsUniversalBridgeLib/Universal Bridge  Arms=3  SnubberResistance=1e5  SnubberCapacitance=inf  Device=IGBT / Diodes  Ron=0.002  Lon=0  ForwardVoltages="[  0  0  ]"  ForwardVoltage=0  GTOparameters=[ 10e-6 , 20e-6 ]  IGBTparameters=[ 1e-6 , 2e-6 ]  Measurements=None  Measurements_2=None  converterType=Rectifier
  Voltage Measurement5 : spsVoltageMeasurementLib/Voltage Measurement  PhasorSimulation=off  OutputType=Complex  PSBequivalent=0
  abc to Alpha-Beta-Zero3 : spsabctoAlphaBetaZeroLib/abc to Alpha-Beta-Zero
  dq0 to Alpha-Beta-Zero : spsdq0toAlphaBetaZeroLib/dq0 to Alpha-Beta-Zero  Alignment=Aligned with phase A axis
  改进PLL1 : Subsystem
  谐波检测 : Subsystem
  a1 : PMIOPort  Side=Right
  b1 : PMIOPort  Port=2  Side=Right
  c1 : PMIOPort  Port=3  Side=Right
  wires:
  Memory/1 -> [PWM]
  PWM2/2(Out1) -> Scope9/1
  Mux7/1 -> Scope4/1, [I2]
  [PWM] -> Universal Bridge1/1
  Subsystem8/3(O3) -> Mux7/3
  Subsystem8/2(O2) -> Mux7/2
  PWM2/1(switch) -> Memory/1
  Mux2/1 -> [Vg]
  Subsystem8/1(O1) -> Sum2/1, Scope2/1, SOGI滤波50Hz3/1, Mux7/1
  Subsystem7/1(O1) -> Mux2/1
  Subsystem7/2(O2) -> Mux2/2
  Subsystem7/3(O3) -> Mux2/3
  [I2b] -> Sum6/2
  Sum4/1 -> " 二阶低通30-1"/1
  Constant1/1 -> Sum4/2
  Mux1/1 -> dq0 to Alpha-Beta-Zero/1
  Sum1/1 -> Gain3/1, Transfer Fcn1/1, Mux5/1
  [wt] -> dq0 to Alpha-Beta-Zero/2
  dq0 to Alpha-Beta-Zero/1 -> Demux5/1
  Sum6/1 -> Gain1/1, Mux5/2, Transfer Fcn2/1
  [I2a] -> Sum1/2
  Sum7/1 -> Sum1/1
  Demux5/1 -> Sum7/2
  Demux5/2 -> Sum8/2
  Sum8/1 -> Sum6/1
  Subsystem9/1(w) -> Mux1/1, Scope3/1
  Voltage Measurement5/1 -> Scope25/1, [Vdc]
  Demux6/2 -> [I2b]
  Demux6/3 -> [I20]
  abc to Alpha-Beta-Zero3/1 -> Demux6/1
  Demux6/1 -> [I2a]
  [I2] -> abc to Alpha-Beta-Zero3/1
  Gain1/1 -> Sum5/2
  Gain3/1 -> Sum/2
  [Vdc] -> Sum4/1
  Alpha-Beta-Zero to dq1/1 -> Subsystem3/1(In2)
  [wt] -> Subsystem3/2(In1), Alpha-Beta-Zero to dq1/2
  Transfer Fcn1/1 -> Sum/1
  Transfer Fcn2/1 -> Sum5/1
  Mux5/1 -> Alpha-Beta-Zero to dq1/1
  Subsystem3/1(Out3) -> Sum/3
  Subsystem3/2(Out1) -> Sum5/3
  [Vg] -> 改进PLL1/1(abc)
  Constant3/1 -> Mux1/2
  [I2bh] -> Sum8/1
  [I2ah] -> Sum7/1
  Constant11/1 -> PV_Cells2/2(T)
  Constant10/1 -> PV_Cells2/1(G)
  Unit Delay3/1 -> PV_Cells2/3(U)
  [Vdc] -> Unit Delay3/1
  Step1/1 -> Subsystem9/Enable
  Saturation1/1 -> Subsystem9/1(di)
  " 二阶低通30-1"/1 -> Saturation1/1
  Step2/1 -> PWM2/Enable
  Sum/1 -> PWM2/1(Via*)
  Sum5/1 -> PWM2/2(Vib*)
  改进PLL1/1(Out2) -> [wt]
  谐波检测/2(Out2) -> [I2bh]
  [wt] -> 谐波检测/2(wt)
  abc/1 -> 谐波检测/1(abc)
  谐波检测/1(Out1) -> [I2ah]
  改进PLL1/2(vab0) -> 谐波检测/3(ab0)
  SOGI滤波50Hz3/1 -> RMS1/1, Sum2/2  "alpha"
  Sum2/1 -> RMS2/1
  RMS1/1 -> Scope/2
  RMS2/1 -> Scope/1
  connections:
  L4/RConn3 -- Subsystem8/LConn3
  C1/LConn1 -- L4/LConn1 -- L3/RConn1
  Subsystem8/LConn1 -- L4/RConn1
  Universal Bridge1/LConn1 -- L3/LConn1
  C1/LConn2 -- L4/LConn2 -- L3/RConn2
  Universal Bridge1/RConn1 -- Voltage Measurement5/LConn1 -- Cpv1/LConn1 -- PV_Cells2/RConn1
  Universal Bridge1/LConn2 -- L3/LConn2
  L4/RConn2 -- Subsystem8/LConn2
  Subsystem7/LConn3 -- b1/RConn1 -- Subsystem8/RConn2
  Universal Bridge1/LConn3 -- L3/LConn3
  L3/RConn3 -- C1/LConn3 -- L4/LConn3
  Subsystem7/LConn1 -- a1/RConn1 -- Subsystem8/RConn1
  Subsystem8/RConn3 -- c1/RConn1 -- Subsystem7/LConn5
  C1/RConn2 -- C1/RConn1 -- C1/RConn3
  Subsystem7/LConn2 -- Subsystem7/LConn4 -- Ground/LConn1 -- Subsystem7/LConn6
  Universal Bridge1/RConn2 -- Voltage Measurement5/LConn2 -- PV_Cells2/RConn2 -- Cpv1/RConn1

== system xieboduoji_13fangzhennow/node3/Subsystem1 ==
  u1 : Inport
  u3 : Inport  Port=2
  u4 : Inport  Port=3
  u5 : Inport  Port=4
  u6 : Inport  Port=5
  u2 : Inport  Port=6
  Pul : DiscretePulseGenerator  PulseType=Time based  Period=5e-5  PulseWidth=40
  RMS1 : Subsystem  TreatAsAtomicUnit=on
  k1 : Outport  VectorParamsAs1DForOutWhenUnconnected=off
  k2 : Outport  Port=2  VectorParamsAs1DForOutWhenUnconnected=off
  k3 : Outport  Port=3  VectorParamsAs1DForOutWhenUnconnected=off
  k4 : Outport  Port=4  VectorParamsAs1DForOutWhenUnconnected=off
  k5 : Outport  Port=5  VectorParamsAs1DForOutWhenUnconnected=off
  k6 : Outport  Port=6  VectorParamsAs1DForOutWhenUnconnected=off
  k7 : Outport  Port=7  VectorParamsAs1DForOutWhenUnconnected=off
  k8 : Outport  Port=8  VectorParamsAs1DForOutWhenUnconnected=off
  k9 : Outport  Port=9  VectorParamsAs1DForOutWhenUnconnected=off
  k10 : Outport  Port=10  VectorParamsAs1DForOutWhenUnconnected=off
  k11 : Outport  Port=11  VectorParamsAs1DForOutWhenUnconnected=off
  k12 : Outport  Port=12  VectorParamsAs1DForOutWhenUnconnected=off
  wires:
  u2/1 -> RMS1/6(u2)
  u6/1 -> RMS1/5(u6)
  u5/1 -> RMS1/4(u5)
  u4/1 -> RMS1/3(u4)
  u3/1 -> RMS1/2(u3)
  u1/1 -> RMS1/1(u1)
  RMS1/12(k12) -> k12/1
  RMS1/11(k11) -> k11/1
  RMS1/10(k10) -> k10/1
  RMS1/9(k9) -> k9/1
  RMS1/8(k8) -> k8/1
  RMS1/7(k7) -> k7/1
  RMS1/6(k6) -> k6/1
  RMS1/5(k5) -> k5/1
  RMS1/4(k4) -> k4/1
  RMS1/3(k3) -> k3/1
  RMS1/2(k2) -> k2/1
  RMS1/1(k1) -> k1/1
  Pul/1 -> RMS1/Trigger

== system xieboduoji_13fangzhennow/node3/Subsystem2 ==
  u1 : Inport
  u3 : Inport  Port=2
  u4 : Inport  Port=3
  u5 : Inport  Port=4
  u6 : Inport  Port=5
  u2 : Inport  Port=6
  Pul : DiscretePulseGenerator  PulseType=Time based  Period=5e-5  PulseWidth=40
  RMS1 : Subsystem  TreatAsAtomicUnit=on
  k1 : Outport  VectorParamsAs1DForOutWhenUnconnected=off
  k2 : Outport  Port=2  VectorParamsAs1DForOutWhenUnconnected=off
  k3 : Outport  Port=3  VectorParamsAs1DForOutWhenUnconnected=off
  k4 : Outport  Port=4  VectorParamsAs1DForOutWhenUnconnected=off
  k5 : Outport  Port=5  VectorParamsAs1DForOutWhenUnconnected=off
  k6 : Outport  Port=6  VectorParamsAs1DForOutWhenUnconnected=off
  k7 : Outport  Port=7  VectorParamsAs1DForOutWhenUnconnected=off
  k8 : Outport  Port=8  VectorParamsAs1DForOutWhenUnconnected=off
  k9 : Outport  Port=9  VectorParamsAs1DForOutWhenUnconnected=off
  k10 : Outport  Port=10  VectorParamsAs1DForOutWhenUnconnected=off
  k11 : Outport  Port=11  VectorParamsAs1DForOutWhenUnconnected=off
  k12 : Outport  Port=12  VectorParamsAs1DForOutWhenUnconnected=off
  wires:
  Pul/1 -> RMS1/Trigger
  RMS1/1(k1) -> k1/1
  RMS1/2(k2) -> k2/1
  RMS1/3(k3) -> k3/1
  RMS1/4(k4) -> k4/1
  RMS1/5(k5) -> k5/1
  RMS1/6(k6) -> k6/1
  RMS1/7(k7) -> k7/1
  RMS1/8(k8) -> k8/1
  RMS1/9(k9) -> k9/1
  RMS1/10(k10) -> k10/1
  RMS1/11(k11) -> k11/1
  RMS1/12(k12) -> k12/1
  u1/1 -> RMS1/1(u1)
  u3/1 -> RMS1/2(u3)
  u4/1 -> RMS1/3(u4)
  u5/1 -> RMS1/4(u5)
  u6/1 -> RMS1/5(u6)
  u2/1 -> RMS1/6(u2)

== system xieboduoji_13fangzhennow/node3/谐波源 ==
  Current Measurement1 : spsCurrentMeasurementLib/Current Measurement  PhasorSimulation=off  OutputType=Complex  PSBequivalent=0
  Demux1 : Demux  Commented=on  Outputs=6
  Demux2 : Demux  Commented=on  Outputs=6
  Display{,1..23} (24 alike) : Display  Commented=on
  Scope : Scope
  Scope1 : Scope  Commented=on
  Scope2 : Scope
  Scope4 : Scope  Commented=on
  Series RLC Branch3 : spsSeriesRLCBranchLib/Series RLC Branch  LConnTagsString=__new0  RConnTagsString=__new0  BranchType=R  Resistance=20  Inductance=0.5e-3  SetiL0=off  InitialCurrent=0  Capacitance=1e-6  Setx0=off  InitialVoltage=0  Measurements=None
  Subsystem1 : Subsystem  Commented=on
  Subsystem2 : Subsystem  Commented=on
  Universal Bridge : spsUniversalBridgeLib/Universal Bridge  Arms=3  SnubberResistance=1e5  SnubberCapacitance=inf  Device=Diodes  Ron=1e-3  Lon=0  ForwardVoltages="[  0  0  ]"  ForwardVoltage=0  GTOparameters=[ 10e-6 , 20e-6 ]  IGBTparameters=[ 1e-6 , 2e-6 ]  Measurements=None  Measurements_2=None  converterType=Rectifier
  Voltage Measure3 : spsVoltageMeasurementLib/Voltage Measurement  PhasorSimulation=off  OutputType=Complex  PSBequivalent=0
  傅里叶分解 : spsFourierLib/Fourier  Freq=50  n=[5 7 11 13 17 19]  InInit=[0, 0]  Ts=0
  A : PMIOPort  Side=Left
  B : PMIOPort  Port=2  Side=Left
  C : PMIOPort  Port=3  Side=Left
  wires:
  Current Measurement1/1 -> 傅里叶分解/1, Scope4/1
  Voltage Measure3/1 -> Scope2/1
  傅里叶分解/1 -> Demux1/1, Scope/1
  傅里叶分解/2 -> Demux2/1, Scope1/1
  Subsystem2/5(k5) -> Display4/1
  Subsystem2/2(k2) -> Display1/1
  Subsystem2/12(k12) -> Display11/1
  Subsystem2/9(k9) -> Display8/1
  Subsystem2/8(k8) -> Display7/1
  Subsystem1/1(k1) -> Display12/1
  Subsystem1/7(k7) -> Display20/1
  Subsystem1/10(k10) -> Display23/1
  Subsystem1/3(k3) -> Display16/1
  Subsystem1/5(k5) -> Display18/1
  Subsystem2/11(k11) -> Display10/1
  Subsystem1/9(k9) -> Display22/1
  Subsystem1/11(k11) -> Display14/1
  Subsystem1/6(k6) -> Display19/1
  Subsystem1/2(k2) -> Display13/1
  Subsystem1/4(k4) -> Display17/1
  Subsystem1/12(k12) -> Display15/1
  Demux2/5 -> Subsystem1/5(u6)
  Demux2/4 -> Subsystem1/4(u5)
  Demux2/2 -> Subsystem1/2(u3)
  Demux2/6 -> Subsystem1/6(u2)
  Demux2/1 -> Subsystem1/1(u1)
  Subsystem2/6(k6) -> Display5/1
  Subsystem2/4(k4) -> Display3/1
  Subsystem2/7(k7) -> Display6/1
  Demux1/6 -> Subsystem2/6(u2)
  Demux1/5 -> Subsystem2/5(u6)
  Demux1/2 -> Subsystem2/2(u3)
  Demux1/4 -> Subsystem2/4(u5)
  Subsystem1/8(k8) -> Display21/1
  Subsystem2/10(k10) -> Display9/1
  Demux1/3 -> Subsystem2/3(u4)
  Subsystem2/3(k3) -> Display2/1
  Demux1/1 -> Subsystem2/1(u1)
  Demux2/3 -> Subsystem1/3(u4)
  Subsystem2/1(k1) -> Display/1
  connections:
  Universal Bridge/LConn3 -- C/RConn1
  Universal Bridge/RConn2 -- Voltage Measure3/LConn2 -- Series RLC Branch3/RConn1
  Universal Bridge/RConn1 -- Series RLC Branch3/LConn1 -- Voltage Measure3/LConn1
  Universal Bridge/LConn2 -- B/RConn1
  Current Measurement1/LConn1 -- Universal Bridge/LConn1
  A/RConn1 -- Current Measurement1/RConn1

== system xieboduoji_13fangzhennow/node4/Subsystem1 ==
  u1 : Inport
  u3 : Inport  Port=2
  u4 : Inport  Port=3
  u5 : Inport  Port=4
  u6 : Inport  Port=5
  u2 : Inport  Port=6
  Pul : DiscretePulseGenerator  PulseType=Time based  Period=5e-5  PulseWidth=40
  RMS1 : Subsystem  TreatAsAtomicUnit=on
  k1 : Outport  VectorParamsAs1DForOutWhenUnconnected=off
  k2 : Outport  Port=2  VectorParamsAs1DForOutWhenUnconnected=off
  k3 : Outport  Port=3  VectorParamsAs1DForOutWhenUnconnected=off
  k4 : Outport  Port=4  VectorParamsAs1DForOutWhenUnconnected=off
  k5 : Outport  Port=5  VectorParamsAs1DForOutWhenUnconnected=off
  k6 : Outport  Port=6  VectorParamsAs1DForOutWhenUnconnected=off
  k7 : Outport  Port=7  VectorParamsAs1DForOutWhenUnconnected=off
  k8 : Outport  Port=8  VectorParamsAs1DForOutWhenUnconnected=off
  k9 : Outport  Port=9  VectorParamsAs1DForOutWhenUnconnected=off
  k10 : Outport  Port=10  VectorParamsAs1DForOutWhenUnconnected=off
  k11 : Outport  Port=11  VectorParamsAs1DForOutWhenUnconnected=off
  k12 : Outport  Port=12  VectorParamsAs1DForOutWhenUnconnected=off
  wires:
  u2/1 -> RMS1/6(u2)
  u6/1 -> RMS1/5(u6)
  u5/1 -> RMS1/4(u5)
  u4/1 -> RMS1/3(u4)
  u3/1 -> RMS1/2(u3)
  u1/1 -> RMS1/1(u1)
  RMS1/12(k12) -> k12/1
  RMS1/11(k11) -> k11/1
  RMS1/10(k10) -> k10/1
  RMS1/9(k9) -> k9/1
  RMS1/8(k8) -> k8/1
  RMS1/7(k7) -> k7/1
  RMS1/6(k6) -> k6/1
  RMS1/5(k5) -> k5/1
  RMS1/4(k4) -> k4/1
  RMS1/3(k3) -> k3/1
  RMS1/2(k2) -> k2/1
  RMS1/1(k1) -> k1/1
  Pul/1 -> RMS1/Trigger

== system xieboduoji_13fangzhennow/node4/Subsystem2 ==
  u1 : Inport
  u3 : Inport  Port=2
  u4 : Inport  Port=3
  u5 : Inport  Port=4
  u6 : Inport  Port=5
  u2 : Inport  Port=6
  Pul : DiscretePulseGenerator  PulseType=Time based  Period=5e-5  PulseWidth=40
  RMS1 : Subsystem  TreatAsAtomicUnit=on
  k1 : Outport  VectorParamsAs1DForOutWhenUnconnected=off
  k2 : Outport  Port=2  VectorParamsAs1DForOutWhenUnconnected=off
  k3 : Outport  Port=3  VectorParamsAs1DForOutWhenUnconnected=off
  k4 : Outport  Port=4  VectorParamsAs1DForOutWhenUnconnected=off
  k5 : Outport  Port=5  VectorParamsAs1DForOutWhenUnconnected=off
  k6 : Outport  Port=6  VectorParamsAs1DForOutWhenUnconnected=off
  k7 : Outport  Port=7  VectorParamsAs1DForOutWhenUnconnected=off
  k8 : Outport  Port=8  VectorParamsAs1DForOutWhenUnconnected=off
  k9 : Outport  Port=9  VectorParamsAs1DForOutWhenUnconnected=off
  k10 : Outport  Port=10  VectorParamsAs1DForOutWhenUnconnected=off
  k11 : Outport  Port=11  VectorParamsAs1DForOutWhenUnconnected=off
  k12 : Outport  Port=12  VectorParamsAs1DForOutWhenUnconnected=off
  wires:
  Pul/1 -> RMS1/Trigger
  RMS1/1(k1) -> k1/1
  RMS1/2(k2) -> k2/1
  RMS1/3(k3) -> k3/1
  RMS1/4(k4) -> k4/1
  RMS1/5(k5) -> k5/1
  RMS1/6(k6) -> k6/1
  RMS1/7(k7) -> k7/1
  RMS1/8(k8) -> k8/1
  RMS1/9(k9) -> k9/1
  RMS1/10(k10) -> k10/1
  RMS1/11(k11) -> k11/1
  RMS1/12(k12) -> k12/1
  u1/1 -> RMS1/1(u1)
  u3/1 -> RMS1/2(u3)
  u4/1 -> RMS1/3(u4)
  u5/1 -> RMS1/4(u5)
  u6/1 -> RMS1/5(u6)
  u2/1 -> RMS1/6(u2)
